simulink model "mvdc_performance_assessment"  (R2018b)
settings: configuration reference "Active" (kept outside this file)
undefined symbols (not defined in the file): DiscIntNeverNeededParam, tS
libraries: misc x8, simulink x1
settings Model: DataDictionary=mvdc_performance_assessment.sldd  Creator=wischnewski  LastModifiedBy=ge34qer

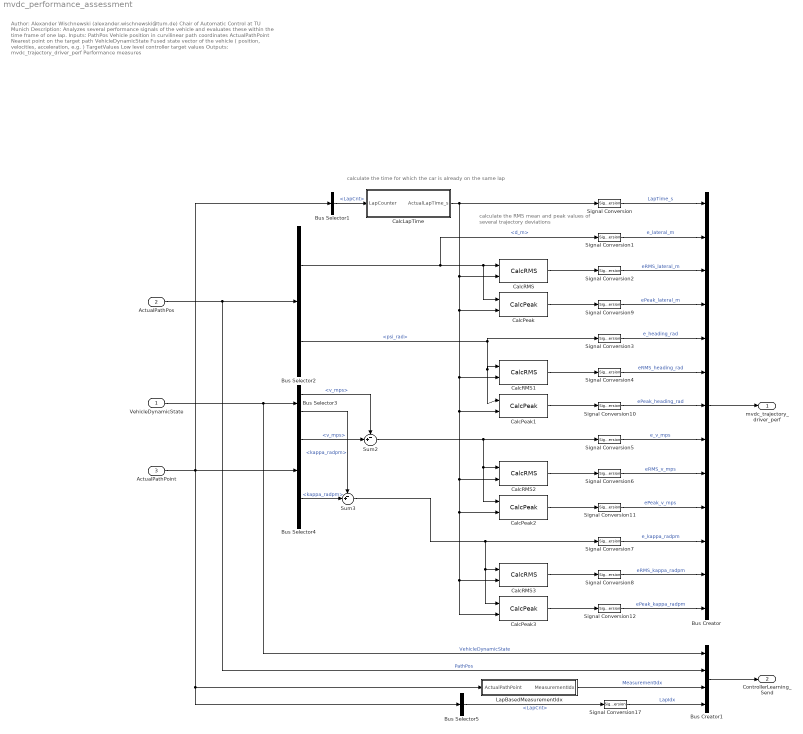
== system mvdc_performance_assessment ==
  note: calculate the RMS mean and peak values
      | of several trajectory deviations
  note: calculate the time for which the car is already on the same lap
  note: Author: Alexander Wischnewski (alexander.wischnewski@tum.de)
      | Chair of Automatic Control at TU Munich
      |
      | Description: Analyzes several performance signals of the vehicle and evaluates these within the time frame of one lap.
      |
      | Inputs:
      | PathPos Vehicle position in curvilinear path coordinates
      | ActualPathPoint Nearest point on the target path
      | VehicleDynamicState Fused state vector of the vehicle ( position, velocities, acceleration, e.g. )
      | TargetValues Low level controller target values
      |
      | Outputs:
      | mvdc_trajectory_driver_perf Performance measures
  VehicleDynamicState : Inport  OutDataTypeStr=Bus: VehicleDynamicState
  ActualPathPos : Inport  Port=2  OutDataTypeStr=Bus: PathPos
  ActualPathPoint : Inport  Port=3  OutDataTypeStr=Bus: PathPoint
  Bus Creator : BusCreator  Inputs=13
  Bus Creator1 : BusCreator  Inputs=4
  Bus Selector1 : BusSelector  OutputSignals=LapCnt
  Bus Selector2 : BusSelector  OutputSignals=d_m,psi_rad
  Bus Selector3 : BusSelector  OutputSignals=v_mps,kappa_radpm
  Bus Selector4 : BusSelector  OutputSignals=v_mps,kappa_radpm
  Bus Selector5 : BusSelector  OutputSignals=LapCnt
  CalcLapTime : Subsystem
  CalcPeak{,1..3} (4 alike) : misc/CalcPeak  SystemSampleTime=-1
  CalcRMS{,1..3} (4 alike) : misc/CalcRMS  SystemSampleTime=-1
  LapBasedMeasurementIdx : Subsystem
  Signal Conversion{,1..12,17} (14 alike) : SignalConversion  OverrideOpt=off
  Sum2 : Sum  Inputs=-+|
  Sum3 : Sum  Inputs=-+|
  mvdc_trajectory_driver_perf : Outport  OutDataTypeStr=Bus: mvdc_trajectory_driver_perf
  ControllerLearning_Send : Outport  Port=2  OutDataTypeStr=Bus: ControllerLearning_Send
  wires:
  Bus Selector4/1 -> Sum2/2  "<v_mps>"
  Bus Selector3/1 -> Sum2/1  "<v_mps>"
  Bus Selector4/2 -> Sum3/2  "<kappa_radpm>"
  Bus Selector3/2 -> Sum3/1  "<kappa_radpm>"
  Sum2/1 -> Signal Conversion5/1, CalcPeak2/1, CalcRMS2/1
  Bus Creator/1 -> mvdc_trajectory_driver_perf/1
  Signal Conversion/1 -> Bus Creator/1  "LapTime_s"
  Signal Conversion1/1 -> Bus Creator/2  "e_lateral_m"
  Signal Conversion2/1 -> Bus Creator/3  "eRMS_lateral_m"
  Signal Conversion3/1 -> Bus Creator/5  "e_heading_rad"
  Signal Conversion4/1 -> Bus Creator/6  "eRMS_heading_rad"
  Signal Conversion5/1 -> Bus Creator/8  "e_v_mps"
  Signal Conversion6/1 -> Bus Creator/9  "eRMS_v_mps"
  Signal Conversion7/1 -> Bus Creator/11  "e_kappa_radpm"
  Signal Conversion8/1 -> Bus Creator/12  "eRMS_kappa_radpm"
  Sum3/1 -> Signal Conversion7/1, CalcRMS3/1, CalcPeak3/1
  CalcRMS/1 -> Signal Conversion2/1
  Signal Conversion9/1 -> Bus Creator/4  "ePeak_lateral_m"
  CalcPeak/1 -> Signal Conversion9/1
  CalcRMS1/1 -> Signal Conversion4/1
  Signal Conversion10/1 -> Bus Creator/7  "ePeak_heading_rad"
  CalcPeak1/1 -> Signal Conversion10/1
  CalcRMS2/1 -> Signal Conversion6/1
  Signal Conversion11/1 -> Bus Creator/10  "ePeak_v_mps"
  CalcPeak2/1 -> Signal Conversion11/1
  CalcRMS3/1 -> Signal Conversion8/1
  Signal Conversion12/1 -> Bus Creator/13  "ePeak_kappa_radpm"
  CalcPeak3/1 -> Signal Conversion12/1
  CalcLapTime/1(ActualLapTime_s) -> Signal Conversion/1, CalcRMS1/2, CalcPeak1/2, CalcRMS2/2, CalcPeak2/2, CalcRMS3/2, CalcPeak3/2, CalcPeak/2, CalcRMS/2
  Bus Selector1/1 -> CalcLapTime/1(LapCounter)  "<LapCnt>"
  Bus Selector2/1 -> Signal Conversion1/1, CalcPeak/1, CalcRMS/1  "<d_m>"
  Bus Selector2/2 -> Signal Conversion3/1, CalcRMS1/1, CalcPeak1/1  "<psi_rad>"
  Bus Creator1/1 -> ControllerLearning_Send/1
  VehicleDynamicState/1 -> Bus Creator1/1, Bus Selector3/1  "VehicleDynamicState"
  ActualPathPos/1 -> Bus Creator1/2, Bus Selector2/1  "PathPos"
  LapBasedMeasurementIdx/1(MeasurementIdx) -> Bus Creator1/3  "MeasurementIdx"
  Bus Selector5/1 -> Signal Conversion17/1  "<LapCnt>"
  Signal Conversion17/1 -> Bus Creator1/4  "LapIdx"
  ActualPathPoint/1 -> Bus Selector4/1, LapBasedMeasurementIdx/1(ActualPathPoint), Bus Selector5/1, Bus Selector1/1

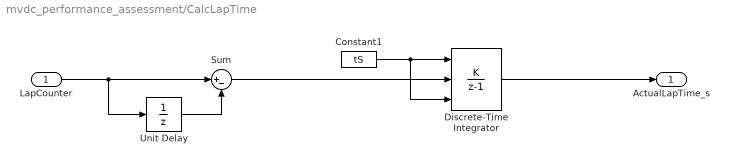
== system mvdc_performance_assessment/CalcLapTime ==
  LapCounter : Inport
  Constant1 : Constant  Value=tS
  Discrete-Time Integrator : DiscreteIntegrator  IntegratorMethod=Accumulation: Forward Euler  ExternalReset=rising  InitialConditionSource=external  SampleTime=-1  ICPrevOutput=DiscIntNeverNeededParam  ICPrevScaledInput=DiscIntNeverNeededParam
  Sum : Sum  Inputs=|+-
  Unit Delay : UnitDelay  SampleTime=-1
  ActualLapTime_s : Outport
  wires:
  LapCounter/1 -> Sum/1, Unit Delay/1
  Sum/1 -> Discrete-Time Integrator/2
  Constant1/1 -> Discrete-Time Integrator/1, Discrete-Time Integrator/3
  Unit Delay/1 -> Sum/2
  Discrete-Time Integrator/1 -> ActualLapTime_s/1

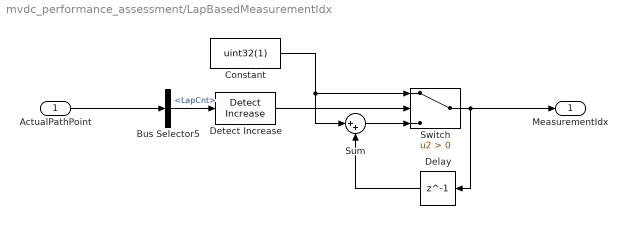
== system mvdc_performance_assessment/LapBasedMeasurementIdx ==
  ActualPathPoint : Inport
  Bus Selector5 : BusSelector  OutputSignals=LapCnt
  Constant : Constant  Value=uint32(1)
  Delay : Delay  DelayLength=1  InitialCondition=uint32(0)
  Detect Increase : simulink/Logic and Bit Operations/Detect Increase  vinit=0.0  OutDataTypeStr=boolean
  Sum : Sum  Inputs=|++
  Switch : Switch  Criteria=u2 > Threshold
  MeasurementIdx : Outport  OutDataTypeStr=uint32
  wires:
  Constant/1 -> Sum/1, Switch/1
  ActualPathPoint/1 -> Bus Selector5/1
  Delay/1 -> Sum/2
  Switch/1 -> MeasurementIdx/1, Delay/1
  Sum/1 -> Switch/3
  Bus Selector5/1 -> Detect Increase/1  "<LapCnt>"
  Detect Increase/1 -> Switch/2
